simulink model "float_sch_PTSD"  (R2020a)
settings: Solver=VariableStepAuto  StartTime=0  StopTime=5  RelTol=1e-3
values from neighbouring files (symbols this model uses):
  buffer_rec = 30    [float_sch_run_PTSD.m]
  diff_th = [50]    [float_sch_run_PTSD.m]
  fs = 30000    [float_sch_run_LocalMaxima_AdaptiveThreshold.m]    (also in float_sch_run_LocalMaxima_HardThreshold.m; float_sch_run_PTSD.m; float_sch_run_Sample_AdaptiveThreshold.m; float_sch_run_Sample_HardThreshold.m)
  PLP = 22    [float_sch_run_PTSD.m]
  refractory = 10^-3    (= 0.001)    [float_sch_run_LocalMaxima_AdaptiveThreshold.m]    (also in float_sch_run_LocalMaxima_HardThreshold.m; float_sch_run_PTSD.m; float_sch_run_Sample_AdaptiveThreshold.m; float_sch_run_Sample_HardThreshold.m)
libraries: simulink x6, dspfdesign x2, dspstat3 x2, dspswit3 x1, hdlsllib x1
settings Model: Creator=sbuccelli  LastModifiedBy=diflo

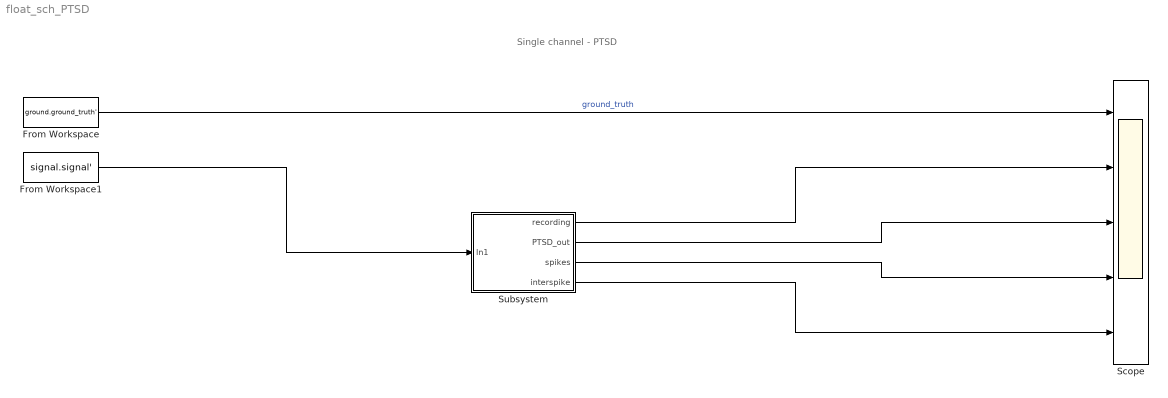
== system float_sch_PTSD ==
  note: Single channel - PTSD
  From Workspace : FromWorkspace  VariableName=ground.ground_truth'  SampleTime=1/fs
  From Workspace1 : FromWorkspace  VariableName=signal.signal'  SampleTime=1/fs
  Scope : Scope  NumInputPorts=5
  Subsystem : Subsystem
  wires:
  From Workspace/1 -> Scope/1  "ground_truth"
  From Workspace1/1 -> Subsystem/1(In1)
  Subsystem/1(recording) -> Scope/2
  Subsystem/2(PTSD_out) -> Scope/3
  Subsystem/3(spikes) -> Scope/4
  Subsystem/4(interspike) -> Scope/5

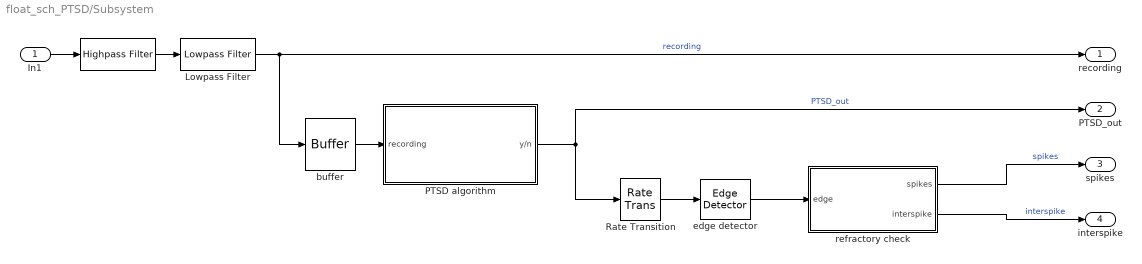
== system float_sch_PTSD/Subsystem ==
  In1 : Inport
  " " : dspfdesign/Highpass Filter  FilterType=IIR  DesignForMinimumOrder=on  FilterOrder=50  StopbandFrequency=1  PassbandFrequency=300  StopbandAttenuation=80  PassbandRipple=0.1  InheritSampleRate=off  SampleRate=fs  SimulateUsing=Interpreted execution  roundingMode=Floor  coeffsDataTypeStr=fixdt(1,16)
  Lowpass Filter : dspfdesign/Lowpass Filter  FilterType=IIR  DesignForMinimumOrder=on  FilterOrder=3  PassbandFrequency=3500  StopbandFrequency=8500  PassbandRipple=0.1  StopbandAttenuation=80  InheritSampleRate=off  SampleRate=fs  SimulateUsing=Interpreted execution  roundingMode=Floor  coeffsDataTypeStr=fixdt(1,16)
  PTSD algorithm : Subsystem
  Rate Transition : RateTransition  OutPortSampleTime=1/fs
  buffer : Buffer  N=buffer_rec  V=buffer_overlap  OutputFrames=off
  edge detector : dspswit3/Edge Detector  InputProcessing=Columns as channels (frame based)
      settings: SourceProductBaseCode=DS
  refractory check : Subsystem
  recording : Outport
  PTSD_out : Outport  Port=2
  spikes : Outport  Port=3
  interspike : Outport  Port=4
  wires:
  buffer/1 -> PTSD algorithm/1(recording)
  " "/1 -> Lowpass Filter/1
  refractory check/2(interspike) -> interspike/1  "interspike"
  edge detector/1 -> refractory check/1(" edge  ")
  Lowpass Filter/1 -> recording/1, buffer/1  "recording"
  PTSD algorithm/1(y/n) -> PTSD_out/1, Rate Transition/1  "PTSD_out"
  Rate Transition/1 -> edge detector/1
  In1/1 -> " "/1
  refractory check/1(" spikes") -> spikes/1  "spikes"

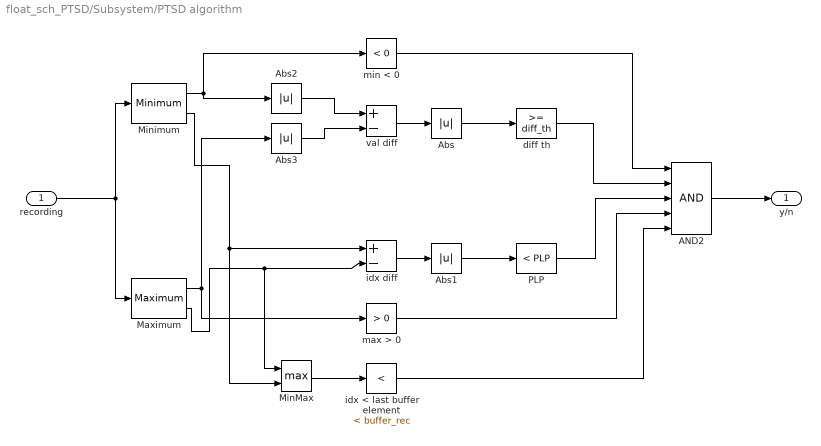
== system float_sch_PTSD/Subsystem/PTSD algorithm ==
  recording : Inport
  AND2 : Logic  Inputs=5  IconShape=distinctive  AllPortsSameDT=off  OutDataTypeStr=boolean
  Abs{,1..3} (4 alike) : Abs
  Maximum : dspstat3/Maximum  operation=maximum  fcn=Value and Index  indexBase=One  operateOver=Each column  Dimension=1  InputProcessing=Columns as channels (frame based)  reset=None  roiEnable=off  roiType=Rectangles  roiPortion=Entire ROI  roiOutput=Individual statistics for each ROI  roiFlag=off  roundingMode=Floor  overflowMode=off  accumDataTypeStr=Inherit: Same as product output  accumLastDataTypeStr=Inherit: Same as product output
  MinMax : MinMax  Function=max  Inputs=2
  Minimum : dspstat3/Minimum  operation=minimum  fcn=Value and Index  indexBase=One  operateOver=Each column  Dimension=1  InputProcessing=Columns as channels (frame based)  reset=None  roiEnable=off  roiType=Rectangles  roiPortion=Entire ROI  roiOutput=Individual statistics for each ROI  roiFlag=off  roundingMode=Floor  overflowMode=off
      settings: SourceProductBaseCode=DS
  PLP : simulink/Logic and Bit Operations/Compare To Constant  relop=<  const=PLP  OutDataTypeStr=boolean
  diff th : simulink/Logic and Bit Operations/Compare To Constant  relop=>=  const=diff_th  OutDataTypeStr=boolean
  idx < last buffer element : simulink/Logic and Bit Operations/Compare To Constant  relop=<  const=buffer_rec  OutDataTypeStr=boolean
  idx diff : Sum  Inputs=+-
  max > 0 : simulink/Logic and Bit Operations/Compare To Constant  relop=>  const=0  OutDataTypeStr=boolean
  min < 0 : simulink/Logic and Bit Operations/Compare To Constant  relop=<  const=0  OutDataTypeStr=boolean
  val diff : Sum  Inputs=+-
  y/n : Outport
  wires:
  Minimum/2 -> MinMax/2, idx diff/1
  Maximum/2 -> MinMax/1, idx diff/2
  val diff/1 -> Abs/1
  Maximum/1 -> Abs3/1, max > 0/1
  Abs1/1 -> PLP/1
  recording/1 -> Maximum/1, Minimum/1
  Abs/1 -> diff th/1
  idx diff/1 -> Abs1/1
  Minimum/1 -> Abs2/1, min < 0/1
  min < 0/1 -> AND2/1
  diff th/1 -> AND2/2
  AND2/1 -> y/n/1
  PLP/1 -> AND2/3
  max > 0/1 -> AND2/4
  Abs2/1 -> val diff/1
  Abs3/1 -> val diff/2
  MinMax/1 -> idx < last buffer element/1
  idx < last buffer element/1 -> AND2/5

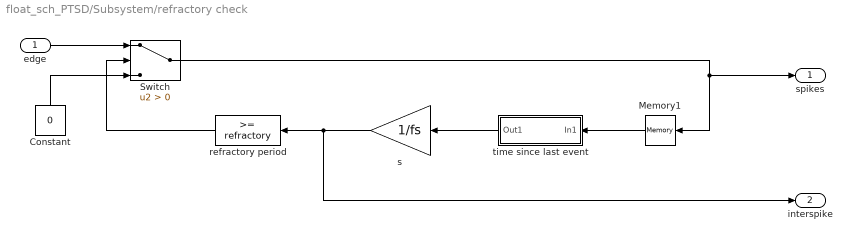
== system float_sch_PTSD/Subsystem/refractory check ==
  " edge  " : Inport
  Constant : Constant  Value=0
  Memory1 : Memory  InheritSampleTime=on
  Switch : Switch  Criteria=u2 > Threshold
  refractory period : simulink/Logic and Bit Operations/Compare To Constant  relop=>=  const=refractory  OutDataTypeStr=boolean
  s : Gain  Gain=1/fs  ParamDataTypeStr=double
  time since last event : Subsystem
  " spikes" : Outport
  interspike : Outport  Port=2
  wires:
  " edge  "/1 -> Switch/1
  Memory1/1 -> time since last event/1(In1)
  time since last event/1(Out1) -> s/1
  Constant/1 -> Switch/3
  s/1 -> refractory period/1, interspike/1
  Switch/1 -> " spikes"/1, Memory1/1
  refractory period/1 -> Switch/2

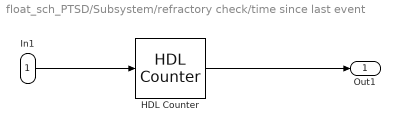
== system float_sch_PTSD/Subsystem/refractory check/time since last event ==
  In1 : Inport
  HDL Counter : hdlsllib/Sources/HDL Counter  CountType=Free running  CountInit=1  CountStep=1  CountMax=25  CountFromType=Initial value  CountFrom=1  CountResetPort=on  CountLoadPort=off  CountEnbPort=off  CountDirPort=off  CountDataType=Unsigned  CountWordLen=32  CountFracLen=0  CountSampTime=1
  Out1 : Outport
  wires:
  In1/1 -> HDL Counter/1
  HDL Counter/1 -> Out1/1
